simulink model "projekt1_8_v2"  (R2016b)
settings: Solver=VariableStepAuto  StartTime=0.0  StopTime=10.0  RelTol=1e-3
values from neighbouring files (symbols this model uses):
  A2 = a1 + 2*a2*u2_ + 3*a3*u2_^2 + 4*a4*u2_^3    (= 0.238125)    [projekt1_5.m]
  B2 = (a1*u2_ + a2*u2_^2 + a3*u2_^3 + a4*u2_^4) - A2*u2_    (= 0.03671875)    [projekt1_5.m]
  K = 3.5    [projekt1.m]    (also in projekt1_5.m)
  T1 = 4    [projekt1.m]    (also in projekt1_5.m)
  T2 = 8    [projekt1.m]    (also in projekt1_5.m)
  Tp = 1    [projekt1.m]    (also in projekt1_5.m)
settings Model: Creator=m  LastModifiedBy=m

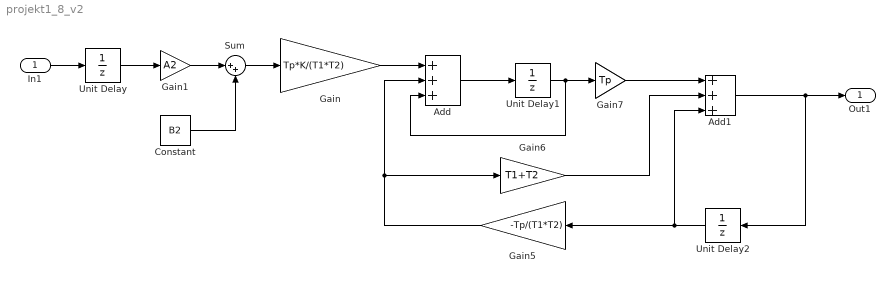
== system projekt1_8_v2 ==
  In1 : Inport
  Add : Sum  Inputs=+++
  Add1 : Sum  Inputs=+++
  Constant : Constant  Value=B2
  Gain : Gain  Gain=Tp*K/(T1*T2)
  Gain1 : Gain  Gain=A2
  Gain5 : Gain  Gain=-Tp/(T1*T2)
  Gain6 : Gain  Gain=T1+T2
  Gain7 : Gain  Gain=Tp
  Sum : Sum  Inputs=|++
  Unit Delay : UnitDelay  SampleTime=-1
  Unit Delay1 : UnitDelay  SampleTime=-1
  Unit Delay2 : UnitDelay  SampleTime=-1
  Out1 : Outport  SignalName=yl(k)
  wires:
  Gain/1 -> Add/1
  Gain5/1 -> Add/2, Gain6/1
  In1/1 -> Unit Delay/1
  Add/1 -> Unit Delay1/1
  Unit Delay1/1 -> Add/3, Gain7/1
  Gain6/1 -> Add1/2
  Gain7/1 -> Add1/1
  Add1/1 -> Unit Delay2/1, Out1/1
  Unit Delay2/1 -> Add1/3, Gain5/1
  Sum/1 -> Gain/1
  Gain1/1 -> Sum/1
  Unit Delay/1 -> Gain1/1
  Constant/1 -> Sum/2
